simulink model "Inertial"  (R2017a)
settings: Solver=VariableStepAuto  StartTime=0.0  StopTime=15  RelTol=1e-3
values from neighbouring files (symbols this model uses):
  c1 = 11    [InertialMatlab.m]
  c2 = 5    [InertialMatlab.m]
  d1 = 0.2    [InertialMatlab.m]
  d2 = 1.0    (= 1)    [InertialMatlab.m]
  J1 = 0.4    [InertialMatlab.m]
  J2 = 1.0    (= 1)    [InertialMatlab.m]
settings Model: Creator=mortenmj  LastModifiedBy=mortenmj

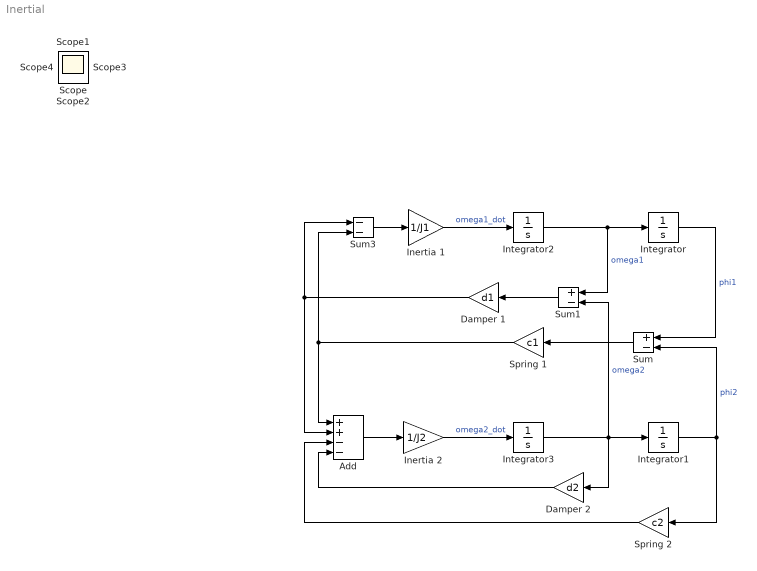
== system Inertial ==
  Add : Sum  Inputs=++--
  Damper 1 : Gain  Gain=d1
  Damper 2 : Gain  Gain=d2
  Inertia 1 : Gain  Gain=1/J1
  Inertia 2 : Gain  Gain=1/J2
  Integrator : Integrator
  Integrator1 : Integrator  InitialCondition=1
  Integrator2 : Integrator
  Integrator3 : Integrator
  Spring 1 : Gain  Gain=c1
  Spring 2 : Gain  Gain=c2
  Sum : Sum  Inputs=+-
  Sum1 : Sum  Inputs=+-
  Sum3 : Sum  Inputs=--
  Scope{,1..4} (5 alike) : Scope
  wires:
  Integrator/1 -> Sum/1  "phi1"
  Integrator2/1 -> Sum1/1, Integrator/1  "omega1"
  Integrator1/1 -> Spring 2/1, Sum/2  "phi2"
  Integrator3/1 -> Integrator1/1, Damper 2/1, Sum1/2  "omega2"
  Inertia 2/1 -> Integrator3/1  "omega2_dot"
  Sum/1 -> Spring 1/1
  Sum1/1 -> Damper 1/1
  Inertia 1/1 -> Integrator2/1  "omega1_dot"
  Sum3/1 -> Inertia 1/1
  Add/1 -> Inertia 2/1
  Damper 2/1 -> Add/4
  Spring 2/1 -> Add/3
  Spring 1/1 -> Sum3/2, Add/1
  Damper 1/1 -> Sum3/1, Add/2
